simulink model "Parallel_n49"  (R2012b)
settings: Solver=VariableStepDiscrete  StartTime=0.0  StopTime=TotalIterations  RelTol=1e-3
values from neighbouring files (symbols this model uses):
  bp = 12    [ConfigValidate.m]
  bpSNMemory = bp    (= 12)    [ConfigValidate.m]
  IterationsOrdering = 4000    [ConfigValidate.m]
  MaxCoordDistance = (abs(max(wx) - min(wx))+abs(max(wy) - min(wy)))^2    [ConfigValidate.m]
  N_limit = 0.01    [ConfigValidate.m]
  nBits = 9    [ConfigValidate.m]
  nBitsNSmemories = (ceil(log2(TotalIterations)))    [ConfigValidate.m]
  S_limit = 1    [ConfigValidate.m]
  SourceNodes = 2000    [ConfigValidate.m]
  ts = 1    [ConfigValidate.m]
  w1 = rand(1,Neurons)    [ConfigValidate.m]
  w2 = rand(1,Neurons)    [ConfigValidate.m]
  wx = zeros(1,Neurons)    [ConfigValidate.m]
  wy = zeros(1,Neurons)    [ConfigValidate.m]
  x1 = rand(SourceNodes,1)    [ConfigValidate.m]
  x2 = rand(SourceNodes,1)    [ConfigValidate.m]
libraries: xbsIndex_r4 x4147, dspsrcs4 x2, dspstat3 x2
(part 11 of 19)

== system Parallel_n49/Neurons/Neuron41 ==
  note: Checking difference between input data and neuron weight
  note: 1. Obtain the distance between this neuron and and winning neuron coordinates
      | 2. Obtaining neighborhood distance: h=exp(-1*(dist²/2S²))
  note: Cooperating Process
  note: Adaptive Process
  note: Updating weights: w(n+1)=wn+N*h*dif
  vX11 : Inport
  vX12 : Inport  Port=2
  S : Inport  Port=3
  N : Inport  Port=4
  MemoryControl : Inport  Port=5
  wx_n1 : Inport  Port=6
  wy_n1 : Inport  Port=7
  wxWinningNeuron : Inport  Port=8
  wyWinningNeuron : Inport  Port=9
  Absolute{,1..3} (4 alike) : xbsIndex_r4/Absolute  precision=Full  arith_type=Unsigned  n_bits=16  bin_pt=14  quantization=Truncate  overflow=Wrap  en=off  latency=dSub_CompetitiveProcess  dbl_ovrd=off  block_type=abs
  CMult : xbsIndex_r4/CMult  const=(2^nBits)/MaxCoordDistance  gui_display_data_type=Fixed-point  const_n_bits=nbGainBlock  const_bin_pt=bpSNMemory  float_type=Single  exp_bits=8  fraction_bits=24  en=off  latency=dGain_CooperatingProcess  precision=User Defined  arith_type=Unsigned  n_bits=nBits  bin_pt=0  quantization="Round  (unbiased: +/- Inf)"  overflow=Wrap  dbl_ovrd=off  use_behavioral_HDL=off  mem_type=Block RAM  pipeline=off  block_type=cmult
  Delay_vX11 : xbsIndex_r4/Delay  rst=off  infoeditControl=Selection of Reset will increase slice count due to use of real FFs and instead of SRLs  en=off  latency=dDelay_CooperatingProcess  dbl_ovrd=off  reg_retiming=off  block_type=delay
  Delay_vX12 : xbsIndex_r4/Delay  rst=off  infoeditControl=Selection of Reset will increase slice count due to use of real FFs and instead of SRLs  en=off  latency=dDelay_CooperatingProcess  dbl_ovrd=off  reg_retiming=off  block_type=delay
  N*h*dif_w1n1 : xbsIndex_r4/Mult  precision=User Defined  arith_type="Signed  (2's comp)"  n_bits=nbMult  bin_pt=bpMult  quantization="Round  (unbiased: +/- Inf)"  overflow=Saturate  en=off  latency=dMult_CooperatingProcess  dbl_ovrd=off  use_behavioral_HDL=off  opt=Speed  use_embedded=on  optimum_pipeline=off  pipeline=on  use_rpm=on  placement_style=Triangular  block_type=mult
  N*h*dif_w2n1 : xbsIndex_r4/Mult  precision=User Defined  arith_type="Signed  (2's comp)"  n_bits=nbMult  bin_pt=bpMult  quantization="Round  (unbiased: +/- Inf)"  overflow=Saturate  en=off  latency=dMult_CooperatingProcess  dbl_ovrd=off  use_behavioral_HDL=off  opt=Speed  use_embedded=on  optimum_pipeline=off  pipeline=on  use_rpm=on  placement_style=Triangular  block_type=mult
  NeighboordFunction_H_n1 : xbsIndex_r4/ROM  depth=2^nBits  initVector=h  distributed_mem=Block RAM  rst=off  init_reg=0  en=on  latency=dMemoryNeighborFunc  gui_display_data_type=Fixed-point  arith_type=Unsigned  n_bits=bp+1  bin_pt=bp  preci_type=Single  exp_width=8  frac_width=24  dbl_ovrd=off  optimize=Area  use_rpm=on  block_type=sprom
  Sum_wxWinning_n1 : xbsIndex_r4/AddSub  mode=Addition  use_carryin=off  use_carryout=off  en=off  latency=dAdd_CooperatingProcess  precision=Full  arith_type=Unsigned  n_bits=nbCoord  bin_pt=bpCoord  quantization=Truncate  overflow=Wrap  dbl_ovrd=off  use_behavioral_HDL=off  hw_selection=Fabric  pipelined=off  block_type=addsub
  Sum_x1n1 : xbsIndex_r4/AddSub  mode=Addition  use_carryin=off  use_carryout=off  en=off  latency=dAdd_CompetitiveProcess  precision=Full  arith_type=Unsigned  n_bits=nb  bin_pt=bp  quantization=Truncate  overflow=Wrap  dbl_ovrd=off  use_behavioral_HDL=off  hw_selection=Fabric  pipelined=off  block_type=addsub
  h*dif_w1n1 : xbsIndex_r4/Mult  precision=User Defined  arith_type="Signed  (2's comp)"  n_bits=nbMult  bin_pt=bpMult  quantization="Round  (unbiased: +/- Inf)"  overflow=Saturate  en=off  latency=dMult_CooperatingProcess  dbl_ovrd=off  use_behavioral_HDL=off  opt=Speed  use_embedded=on  optimum_pipeline=off  pipeline=on  use_rpm=on  placement_style=Triangular  block_type=mult
  h*dif_w1n2 : xbsIndex_r4/Mult  precision=User Defined  arith_type=Unsigned  n_bits=nbCoordMult  bin_pt=bpCoordMult  quantization="Round  (unbiased: +/- Inf)"  overflow=Saturate  en=off  latency=dMult_CooperatingProcess  dbl_ovrd=off  use_behavioral_HDL=off  opt=Speed  use_embedded=on  optimum_pipeline=off  pipeline=on  use_rpm=on  placement_style=Triangular  block_type=mult
  h*dif_w2n1 : xbsIndex_r4/Mult  precision=User Defined  arith_type="Signed  (2's comp)"  n_bits=nbMult  bin_pt=bpMult  quantization="Round  (unbiased: +/- Inf)"  overflow=Saturate  en=off  latency=dMult_CooperatingProcess  dbl_ovrd=off  use_behavioral_HDL=off  opt=Speed  use_embedded=on  optimum_pipeline=off  pipeline=on  use_rpm=on  placement_style=Triangular  block_type=mult
  h_adress1 : xbsIndex_r4/Mult  precision=User Defined  arith_type=Unsigned  n_bits=nb  bin_pt=bp  quantization="Round  (unbiased: +/- Inf)"  overflow=Saturate  en=off  latency=dMultAddress_CooperatingProcess  dbl_ovrd=off  use_behavioral_HDL=off  opt=Speed  use_embedded=on  optimum_pipeline=off  pipeline=on  use_rpm=on  placement_style=Triangular  block_type=mult
  vX12_n1 : xbsIndex_r4/AddSub  mode=Subtraction  use_carryin=off  use_carryout=off  en=off  latency=dSub_CompetitiveProcess  precision=User Defined  arith_type="Signed  (2's comp)"  n_bits=nb  bin_pt=bp  quantization=Truncate  overflow=Wrap  dbl_ovrd=off  use_behavioral_HDL=off  hw_selection=Fabric  pipelined=off  block_type=addsub
  w1n1 : xbsIndex_r4/Register  init=w1(21)  rst=off  en=off  dbl_ovrd=off  block_type=register
  w2n1 : xbsIndex_r4/Register  init=w2(21)  rst=off  en=off  dbl_ovrd=off  block_type=register
  wx+N*h*dif_w1n1 : xbsIndex_r4/AddSub  mode=Addition  use_carryin=off  use_carryout=off  en=off  latency=dSub_CooperatingProcess  precision=User Defined  arith_type="Signed  (2's comp)"  n_bits=nb  bin_pt=bp  quantization=Truncate  overflow=Wrap  dbl_ovrd=off  use_behavioral_HDL=off  hw_selection=Fabric  pipelined=off  block_type=addsub
  wx+N*h*dif_w2n1 : xbsIndex_r4/AddSub  mode=Addition  use_carryin=off  use_carryout=off  en=off  latency=dSub_CooperatingProcess  precision=User Defined  arith_type="Signed  (2's comp)"  n_bits=nb  bin_pt=bp  quantization=Truncate  overflow=Wrap  dbl_ovrd=off  use_behavioral_HDL=off  hw_selection=Fabric  pipelined=off  block_type=addsub
  wx_wxWinning_n1 : xbsIndex_r4/AddSub  mode=Subtraction  use_carryin=off  use_carryout=off  en=off  latency=dSub_CooperatingProcess  precision=User Defined  arith_type="Signed  (2's comp)"  n_bits=nbCoord  bin_pt=bpCoord  quantization=Truncate  overflow=Wrap  dbl_ovrd=off  use_behavioral_HDL=off  hw_selection=Fabric  pipelined=off  block_type=addsub
  wy_wyWinning_n1 : xbsIndex_r4/AddSub  mode=Subtraction  use_carryin=off  use_carryout=off  en=off  latency=dSub_CooperatingProcess  precision=User Defined  arith_type="Signed  (2's comp)"  n_bits=nbCoord  bin_pt=bpCoord  quantization=Truncate  overflow=Wrap  dbl_ovrd=off  use_behavioral_HDL=off  hw_selection=Fabric  pipelined=off  block_type=addsub
  x11_n1 : xbsIndex_r4/AddSub  mode=Subtraction  use_carryin=off  use_carryout=off  en=off  latency=dSub_CompetitiveProcess  precision=User Defined  arith_type="Signed  (2's comp)"  n_bits=nb  bin_pt=bp  quantization=Truncate  overflow=Wrap  dbl_ovrd=off  use_behavioral_HDL=off  hw_selection=Fabric  pipelined=off  block_type=addsub
  w1-n1 : Outport
  w2-n1 : Outport  Port=2
  dist_n1 : Outport  Port=3
  wires:
  wy_wyWinning_n1/1 -> Absolute3/1
  Absolute3/1 -> Sum_wxWinning_n1/2
  Absolute2/1 -> Sum_wxWinning_n1/1
  wx_wxWinning_n1/1 -> Absolute2/1
  h_adress1/1 -> CMult/1
  CMult/1 -> NeighboordFunction_H_n1/1
  S/1 -> h_adress1/1
  wxWinningNeuron/1 -> wx_wxWinning_n1/2
  wy_n1/1 -> wy_wyWinning_n1/1
  wyWinningNeuron/1 -> wy_wyWinning_n1/2
  MemoryControl/1 -> NeighboordFunction_H_n1/2
  h*dif_w2n1/1 -> N*h*dif_w2n1/2
  h*dif_w1n1/1 -> N*h*dif_w1n1/2
  N*h*dif_w2n1/1 -> wx+N*h*dif_w2n1/1
  N*h*dif_w1n1/1 -> wx+N*h*dif_w1n1/2
  wx+N*h*dif_w1n1/1 -> w1n1/1, x11_n1/2
  w1n1/1 -> wx+N*h*dif_w1n1/1, w1-n1/1
  wx+N*h*dif_w2n1/1 -> vX12_n1/2, w2n1/1
  w2n1/1 -> w2-n1/1, wx+N*h*dif_w2n1/2
  NeighboordFunction_H_n1/1 -> h*dif_w2n1/1, h*dif_w1n1/1
  wx_n1/1 -> wx_wxWinning_n1/1
  x11_n1/1 -> Delay_vX11/1, Absolute/1
  vX12_n1/1 -> Delay_vX12/1, Absolute1/1
  Absolute/1 -> Sum_x1n1/1
  Absolute1/1 -> Sum_x1n1/2
  vX12/1 -> vX12_n1/1
  vX11/1 -> x11_n1/1
  Sum_x1n1/1 -> dist_n1/1
  Delay_vX12/1 -> h*dif_w2n1/2
  Delay_vX11/1 -> h*dif_w1n1/2
  Sum_wxWinning_n1/1 -> h*dif_w1n2/2, h*dif_w1n2/1
  h*dif_w1n2/1 -> h_adress1/2
  N/1 -> N*h*dif_w2n1/1, N*h*dif_w1n1/1

== system Parallel_n49/Neurons/Neuron42 ==
  note: Checking difference between input data and neuron weight
  note: 1. Obtain the distance between this neuron and and winning neuron coordinates
      | 2. Obtaining neighborhood distance: h=exp(-1*(dist²/2S²))
  note: Cooperating Process
  note: Adaptive Process
  note: Updating weights: w(n+1)=wn+N*h*dif
  vX11 : Inport
  vX12 : Inport  Port=2
  S : Inport  Port=3
  N : Inport  Port=4
  MemoryControl : Inport  Port=5
  wx_n1 : Inport  Port=6
  wy_n1 : Inport  Port=7
  wxWinningNeuron : Inport  Port=8
  wyWinningNeuron : Inport  Port=9
  Absolute{,1..3} (4 alike) : xbsIndex_r4/Absolute  precision=Full  arith_type=Unsigned  n_bits=16  bin_pt=14  quantization=Truncate  overflow=Wrap  en=off  latency=dSub_CompetitiveProcess  dbl_ovrd=off  block_type=abs
  CMult : xbsIndex_r4/CMult  const=(2^nBits)/MaxCoordDistance  gui_display_data_type=Fixed-point  const_n_bits=nbGainBlock  const_bin_pt=bpSNMemory  float_type=Single  exp_bits=8  fraction_bits=24  en=off  latency=dGain_CooperatingProcess  precision=User Defined  arith_type=Unsigned  n_bits=nBits  bin_pt=0  quantization="Round  (unbiased: +/- Inf)"  overflow=Wrap  dbl_ovrd=off  use_behavioral_HDL=off  mem_type=Block RAM  pipeline=off  block_type=cmult
  Delay_vX11 : xbsIndex_r4/Delay  rst=off  infoeditControl=Selection of Reset will increase slice count due to use of real FFs and instead of SRLs  en=off  latency=dDelay_CooperatingProcess  dbl_ovrd=off  reg_retiming=off  block_type=delay
  Delay_vX12 : xbsIndex_r4/Delay  rst=off  infoeditControl=Selection of Reset will increase slice count due to use of real FFs and instead of SRLs  en=off  latency=dDelay_CooperatingProcess  dbl_ovrd=off  reg_retiming=off  block_type=delay
  N*h*dif_w1n1 : xbsIndex_r4/Mult  precision=User Defined  arith_type="Signed  (2's comp)"  n_bits=nbMult  bin_pt=bpMult  quantization="Round  (unbiased: +/- Inf)"  overflow=Saturate  en=off  latency=dMult_CooperatingProcess  dbl_ovrd=off  use_behavioral_HDL=off  opt=Speed  use_embedded=on  optimum_pipeline=off  pipeline=on  use_rpm=on  placement_style=Triangular  block_type=mult
  N*h*dif_w2n1 : xbsIndex_r4/Mult  precision=User Defined  arith_type="Signed  (2's comp)"  n_bits=nbMult  bin_pt=bpMult  quantization="Round  (unbiased: +/- Inf)"  overflow=Saturate  en=off  latency=dMult_CooperatingProcess  dbl_ovrd=off  use_behavioral_HDL=off  opt=Speed  use_embedded=on  optimum_pipeline=off  pipeline=on  use_rpm=on  placement_style=Triangular  block_type=mult
  NeighboordFunction_H_n1 : xbsIndex_r4/ROM  depth=2^nBits  initVector=h  distributed_mem=Block RAM  rst=off  init_reg=0  en=on  latency=dMemoryNeighborFunc  gui_display_data_type=Fixed-point  arith_type="Signed  (2's comp)"  n_bits=bp+1  bin_pt=bp  preci_type=Single  exp_width=8  frac_width=24  dbl_ovrd=off  optimize=Area  use_rpm=on  block_type=sprom
  Sum_wxWinning_n1 : xbsIndex_r4/AddSub  mode=Addition  use_carryin=off  use_carryout=off  en=off  latency=dAdd_CooperatingProcess  precision=Full  arith_type=Unsigned  n_bits=nbCoord  bin_pt=bpCoord  quantization=Truncate  overflow=Wrap  dbl_ovrd=off  use_behavioral_HDL=off  hw_selection=Fabric  pipelined=off  block_type=addsub
  Sum_x1n1 : xbsIndex_r4/AddSub  mode=Addition  use_carryin=off  use_carryout=off  en=off  latency=dAdd_CompetitiveProcess  precision=Full  arith_type=Unsigned  n_bits=nb  bin_pt=bp  quantization=Truncate  overflow=Wrap  dbl_ovrd=off  use_behavioral_HDL=off  hw_selection=Fabric  pipelined=off  block_type=addsub
  h*dif_w1n1 : xbsIndex_r4/Mult  precision=User Defined  arith_type="Signed  (2's comp)"  n_bits=nbMult  bin_pt=bpMult  quantization="Round  (unbiased: +/- Inf)"  overflow=Saturate  en=off  latency=dMult_CooperatingProcess  dbl_ovrd=off  use_behavioral_HDL=off  opt=Speed  use_embedded=on  optimum_pipeline=off  pipeline=on  use_rpm=on  placement_style=Triangular  block_type=mult
  h*dif_w1n2 : xbsIndex_r4/Mult  precision=User Defined  arith_type=Unsigned  n_bits=nbCoordMult  bin_pt=bpCoordMult  quantization="Round  (unbiased: +/- Inf)"  overflow=Saturate  en=off  latency=dMult_CooperatingProcess  dbl_ovrd=off  use_behavioral_HDL=off  opt=Speed  use_embedded=on  optimum_pipeline=off  pipeline=on  use_rpm=on  placement_style=Triangular  block_type=mult
  h*dif_w2n1 : xbsIndex_r4/Mult  precision=User Defined  arith_type="Signed  (2's comp)"  n_bits=nb  bin_pt=bp  quantization="Round  (unbiased: +/- Inf)"  overflow=Saturate  en=off  latency=dMult_CooperatingProcess  dbl_ovrd=off  use_behavioral_HDL=off  opt=Speed  use_embedded=on  optimum_pipeline=off  pipeline=on  use_rpm=on  placement_style=Triangular  block_type=mult
  h_adress1 : xbsIndex_r4/Mult  precision=User Defined  arith_type=Unsigned  n_bits=nb  bin_pt=bp  quantization="Round  (unbiased: +/- Inf)"  overflow=Saturate  en=off  latency=dMultAddress_CooperatingProcess  dbl_ovrd=off  use_behavioral_HDL=off  opt=Speed  use_embedded=on  optimum_pipeline=off  pipeline=on  use_rpm=on  placement_style=Triangular  block_type=mult
  vX12_n1 : xbsIndex_r4/AddSub  mode=Subtraction  use_carryin=off  use_carryout=off  en=off  latency=dSub_CompetitiveProcess  precision=User Defined  arith_type="Signed  (2's comp)"  n_bits=nb  bin_pt=bp  quantization=Truncate  overflow=Wrap  dbl_ovrd=off  use_behavioral_HDL=off  hw_selection=Fabric  pipelined=off  block_type=addsub
  w1n1 : xbsIndex_r4/Register  init=w1(22)  rst=off  en=off  dbl_ovrd=off  block_type=register
  w2n1 : xbsIndex_r4/Register  init=w2(22)  rst=off  en=off  dbl_ovrd=off  block_type=register
  wx+N*h*dif_w1n1 : xbsIndex_r4/AddSub  mode=Addition  use_carryin=off  use_carryout=off  en=off  latency=dSub_CooperatingProcess  precision=User Defined  arith_type="Signed  (2's comp)"  n_bits=nb  bin_pt=bp  quantization=Truncate  overflow=Wrap  dbl_ovrd=off  use_behavioral_HDL=off  hw_selection=Fabric  pipelined=off  block_type=addsub
  wx+N*h*dif_w2n1 : xbsIndex_r4/AddSub  mode=Addition  use_carryin=off  use_carryout=off  en=off  latency=dSub_CooperatingProcess  precision=User Defined  arith_type="Signed  (2's comp)"  n_bits=nb  bin_pt=bp  quantization=Truncate  overflow=Wrap  dbl_ovrd=off  use_behavioral_HDL=off  hw_selection=Fabric  pipelined=off  block_type=addsub
  wx_wxWinning_n1 : xbsIndex_r4/AddSub  mode=Subtraction  use_carryin=off  use_carryout=off  en=off  latency=dSub_CooperatingProcess  precision=User Defined  arith_type="Signed  (2's comp)"  n_bits=nbCoord  bin_pt=bpCoord  quantization=Truncate  overflow=Wrap  dbl_ovrd=off  use_behavioral_HDL=off  hw_selection=Fabric  pipelined=off  block_type=addsub
  wy_wyWinning_n1 : xbsIndex_r4/AddSub  mode=Subtraction  use_carryin=off  use_carryout=off  en=off  latency=dSub_CooperatingProcess  precision=User Defined  arith_type="Signed  (2's comp)"  n_bits=nbCoord  bin_pt=bpCoord  quantization=Truncate  overflow=Wrap  dbl_ovrd=off  use_behavioral_HDL=off  hw_selection=Fabric  pipelined=off  block_type=addsub
  x11_n1 : xbsIndex_r4/AddSub  mode=Subtraction  use_carryin=off  use_carryout=off  en=off  latency=dSub_CompetitiveProcess  precision=User Defined  arith_type="Signed  (2's comp)"  n_bits=nb  bin_pt=bp  quantization=Truncate  overflow=Wrap  dbl_ovrd=off  use_behavioral_HDL=off  hw_selection=Fabric  pipelined=off  block_type=addsub
  w1-n1 : Outport
  w2-n1 : Outport  Port=2
  dist_n1 : Outport  Port=3
  wires:
  wy_wyWinning_n1/1 -> Absolute3/1
  Absolute3/1 -> Sum_wxWinning_n1/2
  Absolute2/1 -> Sum_wxWinning_n1/1
  wx_wxWinning_n1/1 -> Absolute2/1
  h_adress1/1 -> CMult/1
  CMult/1 -> NeighboordFunction_H_n1/1
  S/1 -> h_adress1/1
  wxWinningNeuron/1 -> wx_wxWinning_n1/2
  wy_n1/1 -> wy_wyWinning_n1/1
  wyWinningNeuron/1 -> wy_wyWinning_n1/2
  MemoryControl/1 -> NeighboordFunction_H_n1/2
  h*dif_w2n1/1 -> N*h*dif_w2n1/2
  h*dif_w1n1/1 -> N*h*dif_w1n1/2
  N*h*dif_w2n1/1 -> wx+N*h*dif_w2n1/1
  N*h*dif_w1n1/1 -> wx+N*h*dif_w1n1/2
  wx+N*h*dif_w1n1/1 -> w1n1/1, x11_n1/2
  w1n1/1 -> wx+N*h*dif_w1n1/1, w1-n1/1
  wx+N*h*dif_w2n1/1 -> vX12_n1/2, w2n1/1
  w2n1/1 -> w2-n1/1, wx+N*h*dif_w2n1/2
  NeighboordFunction_H_n1/1 -> h*dif_w2n1/1, h*dif_w1n1/1
  wx_n1/1 -> wx_wxWinning_n1/1
  x11_n1/1 -> Delay_vX11/1, Absolute/1
  vX12_n1/1 -> Delay_vX12/1, Absolute1/1
  Absolute/1 -> Sum_x1n1/1
  Absolute1/1 -> Sum_x1n1/2
  vX12/1 -> vX12_n1/1
  vX11/1 -> x11_n1/1
  Sum_x1n1/1 -> dist_n1/1
  Delay_vX12/1 -> h*dif_w2n1/2
  Delay_vX11/1 -> h*dif_w1n1/2
  Sum_wxWinning_n1/1 -> h*dif_w1n2/2, h*dif_w1n2/1
  h*dif_w1n2/1 -> h_adress1/2
  N/1 -> N*h*dif_w2n1/1, N*h*dif_w1n1/1

== system Parallel_n49/Neurons/Neuron43 ==
  note: Checking difference between input data and neuron weight
  note: 1. Obtain the distance between this neuron and and winning neuron coordinates
      | 2. Obtaining neighborhood distance: h=exp(-1*(dist²/2S²))
  note: Cooperating Process
  note: Adaptive Process
  note: Updating weights: w(n+1)=wn+N*h*dif
  vX11 : Inport
  vX12 : Inport  Port=2
  S : Inport  Port=3
  N : Inport  Port=4
  MemoryControl : Inport  Port=5
  wx_n1 : Inport  Port=6
  wy_n1 : Inport  Port=7
  wxWinningNeuron : Inport  Port=8
  wyWinningNeuron : Inport  Port=9
  Absolute{,1..3} (4 alike) : xbsIndex_r4/Absolute  precision=Full  arith_type=Unsigned  n_bits=16  bin_pt=14  quantization=Truncate  overflow=Wrap  en=off  latency=dSub_CompetitiveProcess  dbl_ovrd=off  block_type=abs
  CMult : xbsIndex_r4/CMult  const=(2^nBits)/MaxCoordDistance  gui_display_data_type=Fixed-point  const_n_bits=nbGainBlock  const_bin_pt=bpSNMemory  float_type=Single  exp_bits=8  fraction_bits=24  en=off  latency=dGain_CooperatingProcess  precision=User Defined  arith_type=Unsigned  n_bits=nBits  bin_pt=0  quantization="Round  (unbiased: +/- Inf)"  overflow=Wrap  dbl_ovrd=off  use_behavioral_HDL=off  mem_type=Block RAM  pipeline=off  block_type=cmult
  Delay_vX11 : xbsIndex_r4/Delay  rst=off  infoeditControl=Selection of Reset will increase slice count due to use of real FFs and instead of SRLs  en=off  latency=dDelay_CooperatingProcess  dbl_ovrd=off  reg_retiming=off  block_type=delay
  Delay_vX12 : xbsIndex_r4/Delay  rst=off  infoeditControl=Selection of Reset will increase slice count due to use of real FFs and instead of SRLs  en=off  latency=dDelay_CooperatingProcess  dbl_ovrd=off  reg_retiming=off  block_type=delay
  N*h*dif_w1n1 : xbsIndex_r4/Mult  precision=User Defined  arith_type="Signed  (2's comp)"  n_bits=nbMult  bin_pt=bpMult  quantization="Round  (unbiased: +/- Inf)"  overflow=Saturate  en=off  latency=dMult_CooperatingProcess  dbl_ovrd=off  use_behavioral_HDL=off  opt=Speed  use_embedded=on  optimum_pipeline=off  pipeline=on  use_rpm=on  placement_style=Triangular  block_type=mult
  N*h*dif_w2n1 : xbsIndex_r4/Mult  precision=User Defined  arith_type="Signed  (2's comp)"  n_bits=nbMult  bin_pt=bpMult  quantization="Round  (unbiased: +/- Inf)"  overflow=Saturate  en=off  latency=dMult_CooperatingProcess  dbl_ovrd=off  use_behavioral_HDL=off  opt=Speed  use_embedded=on  optimum_pipeline=off  pipeline=on  use_rpm=on  placement_style=Triangular  block_type=mult
  NeighboordFunction_H_n1 : xbsIndex_r4/ROM  depth=2^nBits  initVector=h  distributed_mem=Block RAM  rst=off  init_reg=0  en=on  latency=dMemoryNeighborFunc  gui_display_data_type=Fixed-point  arith_type=Unsigned  n_bits=bp+1  bin_pt=bp  preci_type=Single  exp_width=8  frac_width=24  dbl_ovrd=off  optimize=Area  use_rpm=on  block_type=sprom
  Sum_wxWinning_n1 : xbsIndex_r4/AddSub  mode=Addition  use_carryin=off  use_carryout=off  en=off  latency=dAdd_CooperatingProcess  precision=Full  arith_type=Unsigned  n_bits=nbCoord  bin_pt=bpCoord  quantization=Truncate  overflow=Wrap  dbl_ovrd=off  use_behavioral_HDL=off  hw_selection=Fabric  pipelined=off  block_type=addsub
  Sum_x1n1 : xbsIndex_r4/AddSub  mode=Addition  use_carryin=off  use_carryout=off  en=off  latency=dAdd_CompetitiveProcess  precision=Full  arith_type=Unsigned  n_bits=nb  bin_pt=bp  quantization=Truncate  overflow=Wrap  dbl_ovrd=off  use_behavioral_HDL=off  hw_selection=Fabric  pipelined=off  block_type=addsub
  h*dif_w1n1 : xbsIndex_r4/Mult  precision=User Defined  arith_type="Signed  (2's comp)"  n_bits=nbMult  bin_pt=bpMult  quantization="Round  (unbiased: +/- Inf)"  overflow=Saturate  en=off  latency=dMult_CooperatingProcess  dbl_ovrd=off  use_behavioral_HDL=off  opt=Speed  use_embedded=on  optimum_pipeline=off  pipeline=on  use_rpm=on  placement_style=Triangular  block_type=mult
  h*dif_w1n2 : xbsIndex_r4/Mult  precision=User Defined  arith_type=Unsigned  n_bits=nbCoordMult  bin_pt=bpCoordMult  quantization="Round  (unbiased: +/- Inf)"  overflow=Saturate  en=off  latency=dMult_CooperatingProcess  dbl_ovrd=off  use_behavioral_HDL=off  opt=Speed  use_embedded=on  optimum_pipeline=off  pipeline=on  use_rpm=on  placement_style=Triangular  block_type=mult
  h*dif_w2n1 : xbsIndex_r4/Mult  precision=User Defined  arith_type="Signed  (2's comp)"  n_bits=nbMult  bin_pt=bpMult  quantization="Round  (unbiased: +/- Inf)"  overflow=Saturate  en=off  latency=dMult_CooperatingProcess  dbl_ovrd=off  use_behavioral_HDL=off  opt=Speed  use_embedded=on  optimum_pipeline=off  pipeline=on  use_rpm=on  placement_style=Triangular  block_type=mult
  h_adress1 : xbsIndex_r4/Mult  precision=User Defined  arith_type=Unsigned  n_bits=nb  bin_pt=bp  quantization="Round  (unbiased: +/- Inf)"  overflow=Saturate  en=off  latency=dMultAddress_CooperatingProcess  dbl_ovrd=off  use_behavioral_HDL=off  opt=Speed  use_embedded=on  optimum_pipeline=off  pipeline=on  use_rpm=on  placement_style=Triangular  block_type=mult
  vX12_n1 : xbsIndex_r4/AddSub  mode=Subtraction  use_carryin=off  use_carryout=off  en=off  latency=dSub_CompetitiveProcess  precision=User Defined  arith_type="Signed  (2's comp)"  n_bits=nb  bin_pt=bp  quantization=Truncate  overflow=Wrap  dbl_ovrd=off  use_behavioral_HDL=off  hw_selection=Fabric  pipelined=off  block_type=addsub
  w1n1 : xbsIndex_r4/Register  init=w1(23)  rst=off  en=off  dbl_ovrd=off  block_type=register
  w2n1 : xbsIndex_r4/Register  init=w2(23)  rst=off  en=off  dbl_ovrd=off  block_type=register
  wx+N*h*dif_w1n1 : xbsIndex_r4/AddSub  mode=Addition  use_carryin=off  use_carryout=off  en=off  latency=dSub_CooperatingProcess  precision=User Defined  arith_type="Signed  (2's comp)"  n_bits=nb  bin_pt=bp  quantization=Truncate  overflow=Wrap  dbl_ovrd=off  use_behavioral_HDL=off  hw_selection=Fabric  pipelined=off  block_type=addsub
  wx+N*h*dif_w2n1 : xbsIndex_r4/AddSub  mode=Addition  use_carryin=off  use_carryout=off  en=off  latency=dSub_CooperatingProcess  precision=User Defined  arith_type="Signed  (2's comp)"  n_bits=nb  bin_pt=bp  quantization=Truncate  overflow=Wrap  dbl_ovrd=off  use_behavioral_HDL=off  hw_selection=Fabric  pipelined=off  block_type=addsub
  wx_wxWinning_n1 : xbsIndex_r4/AddSub  mode=Subtraction  use_carryin=off  use_carryout=off  en=off  latency=dSub_CooperatingProcess  precision=User Defined  arith_type="Signed  (2's comp)"  n_bits=nbCoord  bin_pt=bpCoord  quantization=Truncate  overflow=Wrap  dbl_ovrd=off  use_behavioral_HDL=off  hw_selection=Fabric  pipelined=off  block_type=addsub
  wy_wyWinning_n1 : xbsIndex_r4/AddSub  mode=Subtraction  use_carryin=off  use_carryout=off  en=off  latency=dSub_CooperatingProcess  precision=User Defined  arith_type="Signed  (2's comp)"  n_bits=nbCoord  bin_pt=bpCoord  quantization=Truncate  overflow=Wrap  dbl_ovrd=off  use_behavioral_HDL=off  hw_selection=Fabric  pipelined=off  block_type=addsub
  x11_n1 : xbsIndex_r4/AddSub  mode=Subtraction  use_carryin=off  use_carryout=off  en=off  latency=dSub_CompetitiveProcess  precision=User Defined  arith_type="Signed  (2's comp)"  n_bits=nb  bin_pt=bp  quantization=Truncate  overflow=Wrap  dbl_ovrd=off  use_behavioral_HDL=off  hw_selection=Fabric  pipelined=off  block_type=addsub
  w1-n1 : Outport
  w2-n1 : Outport  Port=2
  dist_n1 : Outport  Port=3
  wires:
  wy_wyWinning_n1/1 -> Absolute3/1
  Absolute3/1 -> Sum_wxWinning_n1/2
  Absolute2/1 -> Sum_wxWinning_n1/1
  wx_wxWinning_n1/1 -> Absolute2/1
  h_adress1/1 -> CMult/1
  CMult/1 -> NeighboordFunction_H_n1/1
  S/1 -> h_adress1/1
  wxWinningNeuron/1 -> wx_wxWinning_n1/2
  wy_n1/1 -> wy_wyWinning_n1/1
  wyWinningNeuron/1 -> wy_wyWinning_n1/2
  MemoryControl/1 -> NeighboordFunction_H_n1/2
  h*dif_w2n1/1 -> N*h*dif_w2n1/2
  h*dif_w1n1/1 -> N*h*dif_w1n1/2
  N*h*dif_w2n1/1 -> wx+N*h*dif_w2n1/1
  N*h*dif_w1n1/1 -> wx+N*h*dif_w1n1/2
  wx+N*h*dif_w1n1/1 -> w1n1/1, x11_n1/2
  w1n1/1 -> wx+N*h*dif_w1n1/1, w1-n1/1
  w2n1/1 -> w2-n1/1, wx+N*h*dif_w2n1/2
  NeighboordFunction_H_n1/1 -> h*dif_w2n1/1, h*dif_w1n1/1
  wx_n1/1 -> wx_wxWinning_n1/1
  x11_n1/1 -> Delay_vX11/1, Absolute/1
  vX12_n1/1 -> Delay_vX12/1, Absolute1/1
  Absolute/1 -> Sum_x1n1/1
  Absolute1/1 -> Sum_x1n1/2
  vX12/1 -> vX12_n1/1
  vX11/1 -> x11_n1/1
  Sum_x1n1/1 -> dist_n1/1
  Delay_vX11/1 -> h*dif_w1n1/2
  Delay_vX12/1 -> h*dif_w2n1/2
  wx+N*h*dif_w2n1/1 -> vX12_n1/2, w2n1/1
  Sum_wxWinning_n1/1 -> h*dif_w1n2/2, h*dif_w1n2/1
  h*dif_w1n2/1 -> h_adress1/2
  N/1 -> N*h*dif_w2n1/1, N*h*dif_w1n1/1

== system Parallel_n49/Neurons/Neuron44 ==
  note: Checking difference between input data and neuron weight
  note: 1. Obtain the distance between this neuron and and winning neuron coordinates
      | 2. Obtaining neighborhood distance: h=exp(-1*(dist²/2S²))
  note: Cooperating Process
  note: Adaptive Process
  note: Updating weights: w(n+1)=wn+N*h*dif
  vX11 : Inport
  vX12 : Inport  Port=2
  S : Inport  Port=3
  N : Inport  Port=4
  MemoryControl : Inport  Port=5
  wx_n1 : Inport  Port=6
  wy_n1 : Inport  Port=7
  wxWinningNeuron : Inport  Port=8
  wyWinningNeuron : Inport  Port=9
  Absolute{,1..3} (4 alike) : xbsIndex_r4/Absolute  precision=Full  arith_type=Unsigned  n_bits=16  bin_pt=14  quantization=Truncate  overflow=Wrap  en=off  latency=dSub_CompetitiveProcess  dbl_ovrd=off  block_type=abs
  CMult : xbsIndex_r4/CMult  const=(2^nBits)/MaxCoordDistance  gui_display_data_type=Fixed-point  const_n_bits=nbGainBlock  const_bin_pt=bpSNMemory  float_type=Single  exp_bits=8  fraction_bits=24  en=off  latency=dGain_CooperatingProcess  precision=User Defined  arith_type=Unsigned  n_bits=nBits  bin_pt=0  quantization="Round  (unbiased: +/- Inf)"  overflow=Wrap  dbl_ovrd=off  use_behavioral_HDL=off  mem_type=Block RAM  pipeline=off  block_type=cmult
  Delay_vX11 : xbsIndex_r4/Delay  rst=off  infoeditControl=Selection of Reset will increase slice count due to use of real FFs and instead of SRLs  en=off  latency=dDelay_CooperatingProcess  dbl_ovrd=off  reg_retiming=off  block_type=delay
  Delay_vX12 : xbsIndex_r4/Delay  rst=off  infoeditControl=Selection of Reset will increase slice count due to use of real FFs and instead of SRLs  en=off  latency=dDelay_CooperatingProcess  dbl_ovrd=off  reg_retiming=off  block_type=delay
  N*h*dif_w1n1 : xbsIndex_r4/Mult  precision=User Defined  arith_type="Signed  (2's comp)"  n_bits=nbMult  bin_pt=bpMult  quantization="Round  (unbiased: +/- Inf)"  overflow=Saturate  en=off  latency=dMult_CooperatingProcess  dbl_ovrd=off  use_behavioral_HDL=off  opt=Speed  use_embedded=on  optimum_pipeline=off  pipeline=on  use_rpm=on  placement_style=Triangular  block_type=mult
  N*h*dif_w2n1 : xbsIndex_r4/Mult  precision=User Defined  arith_type="Signed  (2's comp)"  n_bits=nbMult  bin_pt=bpMult  quantization="Round  (unbiased: +/- Inf)"  overflow=Saturate  en=off  latency=dMult_CooperatingProcess  dbl_ovrd=off  use_behavioral_HDL=off  opt=Speed  use_embedded=on  optimum_pipeline=off  pipeline=on  use_rpm=on  placement_style=Triangular  block_type=mult
  NeighboordFunction_H_n1 : xbsIndex_r4/ROM  depth=2^nBits  initVector=h  distributed_mem=Block RAM  rst=off  init_reg=0  en=on  latency=dMemoryNeighborFunc  gui_display_data_type=Fixed-point  arith_type=Unsigned  n_bits=bp+1  bin_pt=bp  preci_type=Single  exp_width=8  frac_width=24  dbl_ovrd=off  optimize=Area  use_rpm=on  block_type=sprom
  Sum_wxWinning_n1 : xbsIndex_r4/AddSub  mode=Addition  use_carryin=off  use_carryout=off  en=off  latency=dAdd_CooperatingProcess  precision=Full  arith_type=Unsigned  n_bits=nbCoord  bin_pt=bpCoord  quantization=Truncate  overflow=Wrap  dbl_ovrd=off  use_behavioral_HDL=off  hw_selection=Fabric  pipelined=off  block_type=addsub
  Sum_x1n1 : xbsIndex_r4/AddSub  mode=Addition  use_carryin=off  use_carryout=off  en=off  latency=dAdd_CompetitiveProcess  precision=Full  arith_type=Unsigned  n_bits=nb  bin_pt=bp  quantization=Truncate  overflow=Wrap  dbl_ovrd=off  use_behavioral_HDL=off  hw_selection=Fabric  pipelined=off  block_type=addsub
  h*dif_w1n1 : xbsIndex_r4/Mult  precision=User Defined  arith_type="Signed  (2's comp)"  n_bits=nbMult  bin_pt=bpMult  quantization="Round  (unbiased: +/- Inf)"  overflow=Saturate  en=off  latency=dMult_CooperatingProcess  dbl_ovrd=off  use_behavioral_HDL=off  opt=Speed  use_embedded=on  optimum_pipeline=off  pipeline=on  use_rpm=on  placement_style=Triangular  block_type=mult
  h*dif_w1n2 : xbsIndex_r4/Mult  precision=User Defined  arith_type=Unsigned  n_bits=nbCoordMult  bin_pt=bpCoordMult  quantization="Round  (unbiased: +/- Inf)"  overflow=Saturate  en=off  latency=dMult_CooperatingProcess  dbl_ovrd=off  use_behavioral_HDL=off  opt=Speed  use_embedded=on  optimum_pipeline=off  pipeline=on  use_rpm=on  placement_style=Triangular  block_type=mult
  h*dif_w2n1 : xbsIndex_r4/Mult  precision=User Defined  arith_type="Signed  (2's comp)"  n_bits=nbMult  bin_pt=bpMult  quantization="Round  (unbiased: +/- Inf)"  overflow=Saturate  en=off  latency=dMult_CooperatingProcess  dbl_ovrd=off  use_behavioral_HDL=off  opt=Speed  use_embedded=on  optimum_pipeline=off  pipeline=on  use_rpm=on  placement_style=Triangular  block_type=mult
  h_adress1 : xbsIndex_r4/Mult  precision=User Defined  arith_type=Unsigned  n_bits=nb  bin_pt=bp  quantization="Round  (unbiased: +/- Inf)"  overflow=Saturate  en=off  latency=dMultAddress_CooperatingProcess  dbl_ovrd=off  use_behavioral_HDL=off  opt=Speed  use_embedded=on  optimum_pipeline=off  pipeline=on  use_rpm=on  placement_style=Triangular  block_type=mult
  vX12_n1 : xbsIndex_r4/AddSub  mode=Subtraction  use_carryin=off  use_carryout=off  en=off  latency=dSub_CompetitiveProcess  precision=User Defined  arith_type="Signed  (2's comp)"  n_bits=nb  bin_pt=bp  quantization=Truncate  overflow=Wrap  dbl_ovrd=off  use_behavioral_HDL=off  hw_selection=Fabric  pipelined=off  block_type=addsub
  w1n1 : xbsIndex_r4/Register  init=w1(24)  rst=off  en=off  dbl_ovrd=off  block_type=register
  w2n1 : xbsIndex_r4/Register  init=w2(24)  rst=off  en=off  dbl_ovrd=off  block_type=register
  wx+N*h*dif_w1n1 : xbsIndex_r4/AddSub  mode=Addition  use_carryin=off  use_carryout=off  en=off  latency=dSub_CooperatingProcess  precision=User Defined  arith_type="Signed  (2's comp)"  n_bits=nb  bin_pt=bp  quantization=Truncate  overflow=Wrap  dbl_ovrd=off  use_behavioral_HDL=off  hw_selection=Fabric  pipelined=off  block_type=addsub
  wx+N*h*dif_w2n1 : xbsIndex_r4/AddSub  mode=Addition  use_carryin=off  use_carryout=off  en=off  latency=dSub_CooperatingProcess  precision=User Defined  arith_type="Signed  (2's comp)"  n_bits=nb  bin_pt=bp  quantization=Truncate  overflow=Wrap  dbl_ovrd=off  use_behavioral_HDL=off  hw_selection=Fabric  pipelined=off  block_type=addsub
  wx_wxWinning_n1 : xbsIndex_r4/AddSub  mode=Subtraction  use_carryin=off  use_carryout=off  en=off  latency=dSub_CooperatingProcess  precision=User Defined  arith_type="Signed  (2's comp)"  n_bits=nbCoord  bin_pt=bpCoord  quantization=Truncate  overflow=Wrap  dbl_ovrd=off  use_behavioral_HDL=off  hw_selection=Fabric  pipelined=off  block_type=addsub
  wy_wyWinning_n1 : xbsIndex_r4/AddSub  mode=Subtraction  use_carryin=off  use_carryout=off  en=off  latency=dSub_CooperatingProcess  precision=User Defined  arith_type="Signed  (2's comp)"  n_bits=nbCoord  bin_pt=bpCoord  quantization=Truncate  overflow=Wrap  dbl_ovrd=off  use_behavioral_HDL=off  hw_selection=Fabric  pipelined=off  block_type=addsub
  x11_n1 : xbsIndex_r4/AddSub  mode=Subtraction  use_carryin=off  use_carryout=off  en=off  latency=dSub_CompetitiveProcess  precision=User Defined  arith_type="Signed  (2's comp)"  n_bits=nb  bin_pt=bp  quantization=Truncate  overflow=Wrap  dbl_ovrd=off  use_behavioral_HDL=off  hw_selection=Fabric  pipelined=off  block_type=addsub
  w1-n1 : Outport
  w2-n1 : Outport  Port=2
  dist_n1 : Outport  Port=3
  wires:
  wy_wyWinning_n1/1 -> Absolute3/1
  Absolute3/1 -> Sum_wxWinning_n1/2
  Absolute2/1 -> Sum_wxWinning_n1/1
  wx_wxWinning_n1/1 -> Absolute2/1
  h_adress1/1 -> CMult/1
  CMult/1 -> NeighboordFunction_H_n1/1
  S/1 -> h_adress1/1
  wxWinningNeuron/1 -> wx_wxWinning_n1/2
  wy_n1/1 -> wy_wyWinning_n1/1
  wyWinningNeuron/1 -> wy_wyWinning_n1/2
  MemoryControl/1 -> NeighboordFunction_H_n1/2
  h*dif_w2n1/1 -> N*h*dif_w2n1/2
  h*dif_w1n1/1 -> N*h*dif_w1n1/2
  N*h*dif_w2n1/1 -> wx+N*h*dif_w2n1/1
  N*h*dif_w1n1/1 -> wx+N*h*dif_w1n1/2
  wx+N*h*dif_w1n1/1 -> w1n1/1, x11_n1/2
  w1n1/1 -> w1-n1/1, wx+N*h*dif_w1n1/1
  w2n1/1 -> w2-n1/1, wx+N*h*dif_w2n1/2
  NeighboordFunction_H_n1/1 -> h*dif_w2n1/1, h*dif_w1n1/1
  wx_n1/1 -> wx_wxWinning_n1/1
  x11_n1/1 -> Delay_vX11/1, Absolute/1
  vX12_n1/1 -> Delay_vX12/1, Absolute1/1
  Absolute/1 -> Sum_x1n1/1
  Absolute1/1 -> Sum_x1n1/2
  vX12/1 -> vX12_n1/1
  vX11/1 -> x11_n1/1
  Sum_x1n1/1 -> dist_n1/1
  Delay_vX11/1 -> h*dif_w1n1/2
  Delay_vX12/1 -> h*dif_w2n1/2
  wx+N*h*dif_w2n1/1 -> vX12_n1/2, w2n1/1
  Sum_wxWinning_n1/1 -> h*dif_w1n2/2, h*dif_w1n2/1
  h*dif_w1n2/1 -> h_adress1/2
  N/1 -> N*h*dif_w2n1/1, N*h*dif_w1n1/1

== system Parallel_n49/Neurons/Neuron45 ==
  note: Checking difference between input data and neuron weight
  note: 1. Obtain the distance between this neuron and and winning neuron coordinates
      | 2. Obtaining neighborhood distance: h=exp(-1*(dist²/2S²))
  note: Cooperating Process
  note: Adaptive Process
  note: Updating weights: w(n+1)=wn+N*h*dif
  vX11 : Inport
  vX12 : Inport  Port=2
  S : Inport  Port=3
  N : Inport  Port=4
  MemoryControl : Inport  Port=5
  wx_n1 : Inport  Port=6
  wy_n1 : Inport  Port=7
  wxWinningNeuron : Inport  Port=8
  wyWinningNeuron : Inport  Port=9
  Absolute{,1..3} (4 alike) : xbsIndex_r4/Absolute  precision=Full  arith_type=Unsigned  n_bits=16  bin_pt=14  quantization=Truncate  overflow=Wrap  en=off  latency=dSub_CompetitiveProcess  dbl_ovrd=off  block_type=abs
  CMult : xbsIndex_r4/CMult  const=(2^nBits)/MaxCoordDistance  gui_display_data_type=Fixed-point  const_n_bits=nbGainBlock  const_bin_pt=bpSNMemory  float_type=Single  exp_bits=8  fraction_bits=24  en=off  latency=dGain_CooperatingProcess  precision=User Defined  arith_type=Unsigned  n_bits=nBits  bin_pt=0  quantization="Round  (unbiased: +/- Inf)"  overflow=Wrap  dbl_ovrd=off  use_behavioral_HDL=off  mem_type=Block RAM  pipeline=off  block_type=cmult
  Delay_vX11 : xbsIndex_r4/Delay  rst=off  infoeditControl=Selection of Reset will increase slice count due to use of real FFs and instead of SRLs  en=off  latency=dDelay_CooperatingProcess  dbl_ovrd=off  reg_retiming=off  block_type=delay
  Delay_vX12 : xbsIndex_r4/Delay  rst=off  infoeditControl=Selection of Reset will increase slice count due to use of real FFs and instead of SRLs  en=off  latency=dDelay_CooperatingProcess  dbl_ovrd=off  reg_retiming=off  block_type=delay
  N*h*dif_w1n1 : xbsIndex_r4/Mult  precision=User Defined  arith_type="Signed  (2's comp)"  n_bits=nbMult  bin_pt=bpMult  quantization="Round  (unbiased: +/- Inf)"  overflow=Saturate  en=off  latency=dMult_CooperatingProcess  dbl_ovrd=off  use_behavioral_HDL=off  opt=Speed  use_embedded=on  optimum_pipeline=off  pipeline=on  use_rpm=on  placement_style=Triangular  block_type=mult
  N*h*dif_w2n1 : xbsIndex_r4/Mult  precision=User Defined  arith_type="Signed  (2's comp)"  n_bits=nbMult  bin_pt=bpMult  quantization="Round  (unbiased: +/- Inf)"  overflow=Saturate  en=off  latency=dMult_CooperatingProcess  dbl_ovrd=off  use_behavioral_HDL=off  opt=Speed  use_embedded=on  optimum_pipeline=off  pipeline=on  use_rpm=on  placement_style=Triangular  block_type=mult
  NeighboordFunction_H_n1 : xbsIndex_r4/ROM  depth=2^nBits  initVector=h  distributed_mem=Block RAM  rst=off  init_reg=0  en=on  latency=dMemoryNeighborFunc  gui_display_data_type=Fixed-point  arith_type=Unsigned  n_bits=bp+1  bin_pt=bp  preci_type=Single  exp_width=8  frac_width=24  dbl_ovrd=off  optimize=Area  use_rpm=on  block_type=sprom
  Sum_wxWinning_n1 : xbsIndex_r4/AddSub  mode=Addition  use_carryin=off  use_carryout=off  en=off  latency=dAdd_CooperatingProcess  precision=Full  arith_type=Unsigned  n_bits=nbCoord  bin_pt=bpCoord  quantization=Truncate  overflow=Wrap  dbl_ovrd=off  use_behavioral_HDL=off  hw_selection=Fabric  pipelined=off  block_type=addsub
  Sum_x1n1 : xbsIndex_r4/AddSub  mode=Addition  use_carryin=off  use_carryout=off  en=off  latency=dAdd_CompetitiveProcess  precision=Full  arith_type=Unsigned  n_bits=nb  bin_pt=bp  quantization=Truncate  overflow=Wrap  dbl_ovrd=off  use_behavioral_HDL=off  hw_selection=Fabric  pipelined=off  block_type=addsub
  h*dif_w1n1 : xbsIndex_r4/Mult  precision=User Defined  arith_type="Signed  (2's comp)"  n_bits=nbMult  bin_pt=bpMult  quantization="Round  (unbiased: +/- Inf)"  overflow=Saturate  en=off  latency=dMult_CooperatingProcess  dbl_ovrd=off  use_behavioral_HDL=off  opt=Speed  use_embedded=on  optimum_pipeline=off  pipeline=on  use_rpm=on  placement_style=Triangular  block_type=mult
  h*dif_w1n2 : xbsIndex_r4/Mult  precision=User Defined  arith_type=Unsigned  n_bits=nbCoordMult  bin_pt=bpCoordMult  quantization="Round  (unbiased: +/- Inf)"  overflow=Saturate  en=off  latency=dMult_CooperatingProcess  dbl_ovrd=off  use_behavioral_HDL=off  opt=Speed  use_embedded=on  optimum_pipeline=off  pipeline=on  use_rpm=on  placement_style=Triangular  block_type=mult
  h*dif_w2n1 : xbsIndex_r4/Mult  precision=User Defined  arith_type="Signed  (2's comp)"  n_bits=nbMult  bin_pt=bpMult  quantization="Round  (unbiased: +/- Inf)"  overflow=Saturate  en=off  latency=dMult_CooperatingProcess  dbl_ovrd=off  use_behavioral_HDL=off  opt=Speed  use_embedded=on  optimum_pipeline=off  pipeline=on  use_rpm=on  placement_style=Triangular  block_type=mult
  h_adress1 : xbsIndex_r4/Mult  precision=User Defined  arith_type=Unsigned  n_bits=nb  bin_pt=bp  quantization="Round  (unbiased: +/- Inf)"  overflow=Saturate  en=off  latency=dMultAddress_CooperatingProcess  dbl_ovrd=off  use_behavioral_HDL=off  opt=Speed  use_embedded=on  optimum_pipeline=off  pipeline=on  use_rpm=on  placement_style=Triangular  block_type=mult
  vX12_n1 : xbsIndex_r4/AddSub  mode=Subtraction  use_carryin=off  use_carryout=off  en=off  latency=dSub_CompetitiveProcess  precision=User Defined  arith_type="Signed  (2's comp)"  n_bits=nb  bin_pt=bp  quantization=Truncate  overflow=Wrap  dbl_ovrd=off  use_behavioral_HDL=off  hw_selection=Fabric  pipelined=off  block_type=addsub
  w1n1 : xbsIndex_r4/Register  init=w1(25)  rst=off  en=off  dbl_ovrd=off  block_type=register
  w2n1 : xbsIndex_r4/Register  init=w2(25)  rst=off  en=off  dbl_ovrd=off  block_type=register
  wx+N*h*dif_w1n1 : xbsIndex_r4/AddSub  mode=Addition  use_carryin=off  use_carryout=off  en=off  latency=dSub_CooperatingProcess  precision=User Defined  arith_type="Signed  (2's comp)"  n_bits=nb  bin_pt=bp  quantization=Truncate  overflow=Wrap  dbl_ovrd=off  use_behavioral_HDL=off  hw_selection=Fabric  pipelined=off  block_type=addsub
  wx+N*h*dif_w2n1 : xbsIndex_r4/AddSub  mode=Addition  use_carryin=off  use_carryout=off  en=off  latency=dSub_CooperatingProcess  precision=User Defined  arith_type="Signed  (2's comp)"  n_bits=nb  bin_pt=bp  quantization=Truncate  overflow=Wrap  dbl_ovrd=off  use_behavioral_HDL=off  hw_selection=Fabric  pipelined=off  block_type=addsub
  wx_wxWinning_n1 : xbsIndex_r4/AddSub  mode=Subtraction  use_carryin=off  use_carryout=off  en=off  latency=dSub_CooperatingProcess  precision=User Defined  arith_type="Signed  (2's comp)"  n_bits=nbCoord  bin_pt=bpCoord  quantization=Truncate  overflow=Wrap  dbl_ovrd=off  use_behavioral_HDL=off  hw_selection=Fabric  pipelined=off  block_type=addsub
  wy_wyWinning_n1 : xbsIndex_r4/AddSub  mode=Subtraction  use_carryin=off  use_carryout=off  en=off  latency=dSub_CooperatingProcess  precision=User Defined  arith_type="Signed  (2's comp)"  n_bits=nbCoord  bin_pt=bpCoord  quantization=Truncate  overflow=Wrap  dbl_ovrd=off  use_behavioral_HDL=off  hw_selection=Fabric  pipelined=off  block_type=addsub
  x11_n1 : xbsIndex_r4/AddSub  mode=Subtraction  use_carryin=off  use_carryout=off  en=off  latency=dSub_CompetitiveProcess  precision=User Defined  arith_type="Signed  (2's comp)"  n_bits=nb  bin_pt=bp  quantization=Truncate  overflow=Wrap  dbl_ovrd=off  use_behavioral_HDL=off  hw_selection=Fabric  pipelined=off  block_type=addsub
  w1-n1 : Outport
  w2-n1 : Outport  Port=2
  dist_n1 : Outport  Port=3
  wires:
  wy_wyWinning_n1/1 -> Absolute3/1
  Absolute3/1 -> Sum_wxWinning_n1/2
  Absolute2/1 -> Sum_wxWinning_n1/1
  wx_wxWinning_n1/1 -> Absolute2/1
  h_adress1/1 -> CMult/1
  CMult/1 -> NeighboordFunction_H_n1/1
  S/1 -> h_adress1/1
  wxWinningNeuron/1 -> wx_wxWinning_n1/2
  wy_n1/1 -> wy_wyWinning_n1/1
  wyWinningNeuron/1 -> wy_wyWinning_n1/2
  MemoryControl/1 -> NeighboordFunction_H_n1/2
  h*dif_w2n1/1 -> N*h*dif_w2n1/2
  h*dif_w1n1/1 -> N*h*dif_w1n1/2
  N*h*dif_w2n1/1 -> wx+N*h*dif_w2n1/1
  N*h*dif_w1n1/1 -> wx+N*h*dif_w1n1/2
  wx+N*h*dif_w1n1/1 -> w1n1/1, x11_n1/2
  w1n1/1 -> w1-n1/1, wx+N*h*dif_w1n1/1
  wx+N*h*dif_w2n1/1 -> vX12_n1/2, w2n1/1
  w2n1/1 -> w2-n1/1, wx+N*h*dif_w2n1/2
  NeighboordFunction_H_n1/1 -> h*dif_w2n1/1, h*dif_w1n1/1
  wx_n1/1 -> wx_wxWinning_n1/1
  x11_n1/1 -> Delay_vX11/1, Absolute/1
  vX12_n1/1 -> Delay_vX12/1, Absolute1/1
  Absolute/1 -> Sum_x1n1/1
  Absolute1/1 -> Sum_x1n1/2
  vX12/1 -> vX12_n1/1
  vX11/1 -> x11_n1/1
  Sum_x1n1/1 -> dist_n1/1
  Delay_vX11/1 -> h*dif_w1n1/2
  Delay_vX12/1 -> h*dif_w2n1/2
  h*dif_w1n2/1 -> h_adress1/2
  Sum_wxWinning_n1/1 -> h*dif_w1n2/2, h*dif_w1n2/1
  N/1 -> N*h*dif_w2n1/1, N*h*dif_w1n1/1
